simulink subsystem "PGAx50"  (R2025b)
settings: Solver=VariableStepAuto  StartTime=0.0  StopTime=10.0  RelTol=1e-3
undefined symbols (not defined in the file or in its folder): Gain, Ra_dse, Rb_dse
libraries: fl_lib x2, ee_lib x1
settings Model: Creator=elias  LastModifiedBy=elias

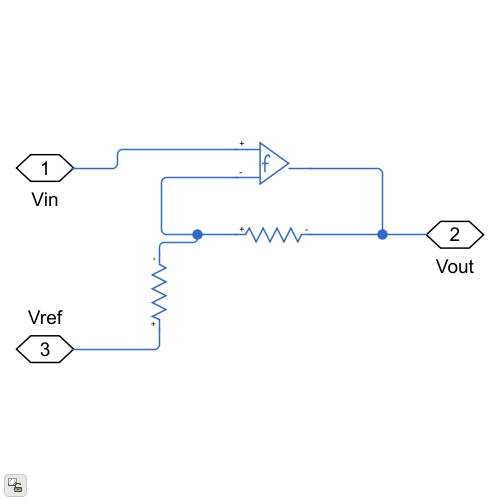
[thumbnail: Simulink's stored preview of the top-level diagram]
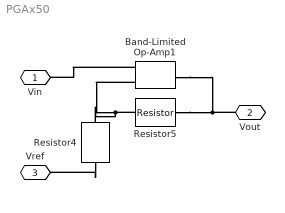
== system PGAx50 ==
  Band-Limited Op-Amp1 : ee_lib/Integrated Circuits/Band-Limited Op-Amp  A=Gain  Rin=Rin Ohm  Rout=Rout Ohm  Vmin=Vmin V  Vmax=Vmax V  Vdotmax=SR V/s  f=BW Hz  V0=0 V
  Resistor4 : fl_lib/Electrical/Electrical Elements/Resistor  R=Ra_dse Ohm  i_specify=off  i_priority=None  i=0 A  i_nominal_specify=off  i_nominal_value=1  i_nominal_unit=A  v_specify=off  v_priority=None  v=0 V  v_nominal_specify=off  v_nominal_value=1  v_nominal_unit=V
  Resistor5 : fl_lib/Electrical/Electrical Elements/Resistor  R=Rb_dse Ohm  i_specify=off  i_priority=None  i=0 A  i_nominal_specify=off  i_nominal_value=1  i_nominal_unit=A  v_specify=off  v_priority=None  v=0 V  v_nominal_specify=off  v_nominal_value=1  v_nominal_unit=V
  Vin : PMIOPort  Side=Left
  Vout : PMIOPort  Port=2  Side=Right
  Vref : PMIOPort  Port=3  Side=Right
  connections:
  Resistor5/RConn1 -- Vout/RConn1 -- Band-Limited Op-Amp1/RConn1
  Resistor4/RConn1 -- Resistor5/LConn1 -- Band-Limited Op-Amp1/LConn2
  Band-Limited Op-Amp1/LConn1 -- Vin/RConn1
  Resistor4/LConn1 -- Vref/RConn1
